simulink model "ex4"  (R2024b)
settings: Solver=FixedStepAuto  StartTime=0.0  StopTime=60  FixedStep=Ts  RelTol=1e-3
undefined symbols (not defined in the file or in its folder): k1, k2, k3, qi
libraries: robotmobilelib x1
settings Model: Creator=fiore  LastModifiedBy=fiore

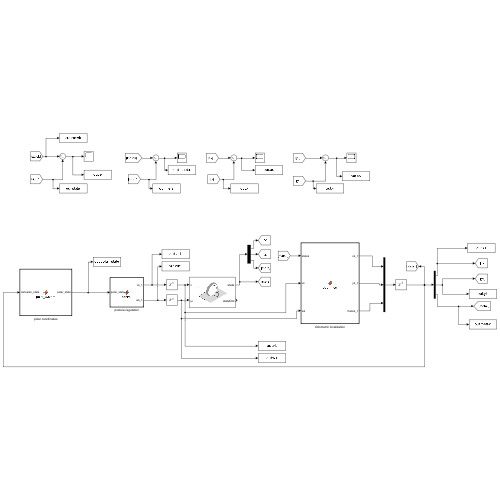
[thumbnail: Simulink's stored preview of the top-level diagram]
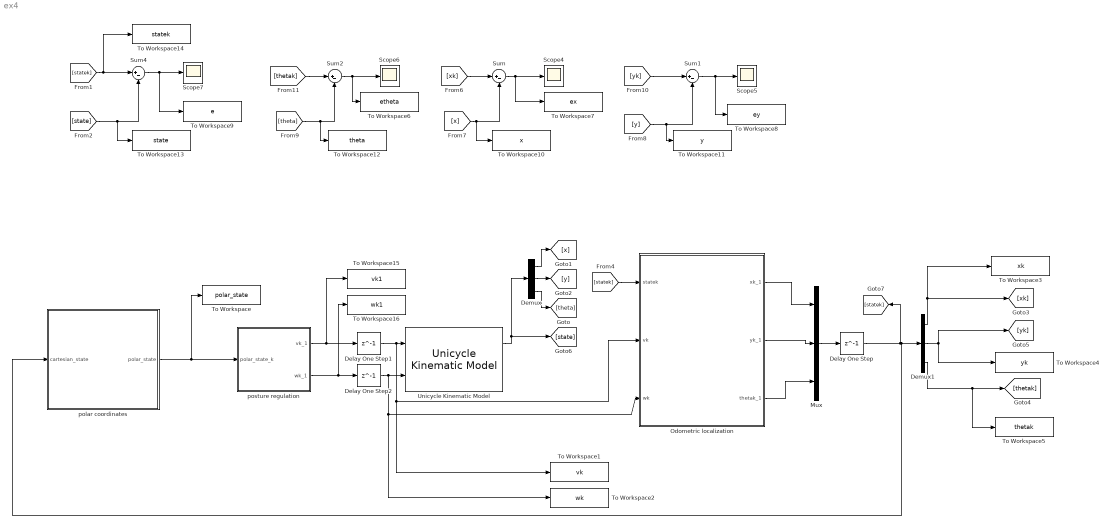
== system ex4 ==
  Delay One Step : Delay  DelayLength=1  InitialCondition=qi
  Delay One Step1 : Delay  DelayLength=1  InitialCondition=0
  Delay One Step2 : Delay  DelayLength=1  InitialCondition=0
  Demux : Demux  Outputs=3
  Demux1 : Demux  Outputs=3
  Mux : Mux  Inputs=3
  Odometric localization : MATLAB Function  TreatAsAtomicUnit=on
  Scope{4..7} (4 alike) : Scope
  Sum{,1..2,4} (4 alike) : Sum  Inputs=|+-
  To Workspace : ToWorkspace  VariableName=polar_state  SaveFormat=Timeseries  SampleTime=-1
  To Workspace1 : ToWorkspace  VariableName=vk  SaveFormat=Timeseries  SampleTime=-1
  To Workspace10 : ToWorkspace  VariableName=x  SaveFormat=Timeseries  SampleTime=-1
  To Workspace11 : ToWorkspace  VariableName=y  SaveFormat=Timeseries  SampleTime=-1
  To Workspace12 : ToWorkspace  VariableName=theta  SaveFormat=Timeseries  SampleTime=-1
  To Workspace13 : ToWorkspace  VariableName=state  SaveFormat=Timeseries  SampleTime=-1
  To Workspace14 : ToWorkspace  VariableName=statek  SaveFormat=Timeseries  SampleTime=-1
  To Workspace15 : ToWorkspace  VariableName=vk1  SaveFormat=Timeseries  SampleTime=-1
  To Workspace16 : ToWorkspace  VariableName=wk1  SaveFormat=Timeseries  SampleTime=-1
  To Workspace2 : ToWorkspace  VariableName=wk  SaveFormat=Timeseries  SampleTime=-1
  To Workspace3 : ToWorkspace  VariableName=xk  SaveFormat=Timeseries  SampleTime=-1
  To Workspace4 : ToWorkspace  VariableName=yk  SaveFormat=Timeseries  SampleTime=-1
  To Workspace5 : ToWorkspace  VariableName=thetak  SaveFormat=Timeseries  SampleTime=-1
  To Workspace6 : ToWorkspace  VariableName=etheta  SaveFormat=Timeseries  SampleTime=-1
  To Workspace7 : ToWorkspace  VariableName=ex  SaveFormat=Timeseries  SampleTime=-1
  To Workspace8 : ToWorkspace  VariableName=ey  SaveFormat=Timeseries  SampleTime=-1
  To Workspace9 : ToWorkspace  VariableName=e  SaveFormat=Timeseries  SampleTime=-1
  Unicycle Kinematic Model : robotmobilelib/Unicycle Kinematic Model  VehicleInputs=Vehicle Speed & Heading Angular Velocity  WheelRadius=0.05  WheelSpeedRange=[-Inf Inf]  InitialState=qi  SimulateUsing=Interpreted execution
  polar coordinates : MATLAB Function  TreatAsAtomicUnit=on
  posture regulation : MATLAB Function  TreatAsAtomicUnit=on
  wires:
  Odometric localization/2(yk_1) -> Mux/2
  Odometric localization/3(thetak_1) -> Mux/3
  Odometric localization/1(xk_1) -> Mux/1
  Mux/1 -> Delay One Step/1
  polar coordinates/1(polar_state) -> To Workspace/1, posture regulation/1(polar_state_k)
  Unicycle Kinematic Model/1 -> Demux/1, [state]
  Demux/3 -> [theta]
  Sum/1 -> To Workspace7/1, Scope4/1
  Sum2/1 -> To Workspace6/1, Scope6/1
  [y] -> To Workspace11/1, Sum1/2
  [theta] -> To Workspace12/1, Sum2/2
  [yk] -> Sum1/1
  [x] -> To Workspace10/1, Sum/2
  [thetak] -> Sum2/1
  [xk] -> Sum/1
  Sum1/1 -> To Workspace8/1, Scope5/1
  Demux/1 -> [x]
  Demux/2 -> [y]
  Demux1/1 -> To Workspace3/1, [xk]
  Demux1/3 -> To Workspace5/1, [thetak]
  Demux1/2 -> To Workspace4/1, [yk]
  posture regulation/2(wk_1) -> To Workspace16/1, Delay One Step2/1
  posture regulation/1(vk_1) -> To Workspace15/1, Delay One Step1/1
  [state] -> To Workspace13/1, Sum4/2
  [statek] -> To Workspace14/1, Sum4/1
  Sum4/1 -> To Workspace9/1, Scope7/1
  Delay One Step/1 -> Demux1/1, polar coordinates/1(cartesian_state), [statek]
  [statek] -> Odometric localization/1(statek)
  Delay One Step1/1 -> To Workspace1/1, Odometric localization/2(vk), Unicycle Kinematic Model/1
  Delay One Step2/1 -> To Workspace2/1, Odometric localization/3(wk), Unicycle Kinematic Model/2

== matlab function ex4/posture regulation ==
  data: polar_state_k input; vk_1 output; wk_1 output; k1 parameter; k2 parameter; k3 parameter
function [vk_1, wk_1] = control(polar_state_k, k1, k2, k3)

rho = polar_state_k(1);
gamma = polar_state_k(2);
delta = polar_state_k(3);

vk_1 = k1*rho*cos(gamma);
wk_1 = k2*gamma + k1*sin(gamma)*cos(gamma)*(1 + k3*delta/gamma);

end

== matlab function ex4/polar coordinates ==
  data: cartesian_state input; polar_state output
function polar_state  = polar_system(cartesian_state)

x = cartesian_state(1);
y = cartesian_state(2);
theta = cartesian_state(3);

rho = sqrt(x^2 + y^2);
gamma = atan2(y,x) - theta + pi;
delta = gamma + theta;

polar_state = [rho, gamma, delta]';
end

== matlab function ex4/Odometric localization ==
  data: statek input; xk_1 output; yk_1 output; thetak_1 output; vk input; wk input; Ts parameter
function [xk_1, yk_1, thetak_1] = odom_loc(statek, vk, wk, Ts)

xk = statek(1);
yk = statek(2);
thetak = statek(3);

xk_1 =  xk + vk*Ts*cos(thetak + wk*Ts/2);
yk_1 = yk + vk*Ts*sin(thetak + wk*Ts/2);
thetak_1 = thetak + wk*Ts;

end
